simulink model "varParam_laplace"  (R2022b)
settings: Solver=VariableStepAuto  StartTime=0.0  StopTime=10.0  MaxStep=1e-3  MinStep=1e-4  RelTol=1e-3
settings Model: Creator=yeyi5  LastModifiedBy=yeyi5
settings DataIOCC: ReturnWorkspaceOutputs=off

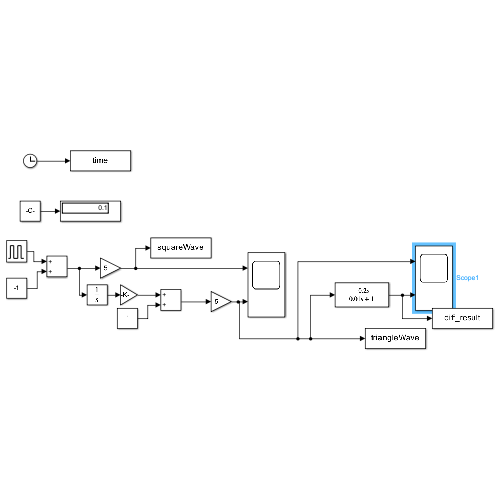
[thumbnail: Simulink's stored preview of the top-level diagram]
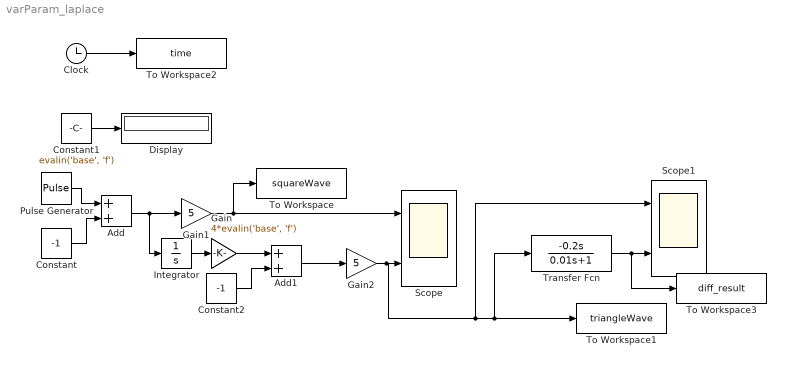
== system varParam_laplace ==
  Add : Sum
  Add1 : Sum
  Clock : Clock
  Constant : Constant  Value=-1
  Constant1 : Constant  Value=evalin('base', 'f')
  Constant2 : Constant  Value=-1
  Display : Display
  Gain : Gain  Gain=4*evalin('base', 'f')
  Gain1 : Gain  Gain=5
  Gain2 : Gain  Gain=5
  Integrator : Integrator
  Pulse Generator : DiscretePulseGenerator  PulseType=Time based  Amplitude=2  Period=evalin('base', '1/f')  PulseWidth=50
  Scope : Scope  NumInputPorts=2
  Scope1 : Scope  NumInputPorts=2
  To Workspace : ToWorkspace  VariableName=squareWave  SampleTime=-1
  To Workspace1 : ToWorkspace  VariableName=triangleWave  SampleTime=-1
  To Workspace2 : ToWorkspace  VariableName=time  SampleTime=-1
  To Workspace3 : ToWorkspace  VariableName=diff_result  SampleTime=-1
  Transfer Fcn : TransferFcn  Numerator=[-0.2, 0]  Denominator=[0.01, 1]
  wires:
  Gain2/1 -> Scope1/1, Transfer Fcn/1, To Workspace1/1, Scope/2
  Constant2/1 -> Add1/2
  Clock/1 -> To Workspace2/1
  Gain1/1 -> To Workspace/1, Scope/1
  Constant1/1 -> Display/1
  Add/1 -> Gain1/1, Integrator/1
  Gain/1 -> Add1/1
  Integrator/1 -> Gain/1
  Pulse Generator/1 -> Add/1
  Constant/1 -> Add/2
  Add1/1 -> Gain2/1
  Transfer Fcn/1 -> To Workspace3/1, Scope1/2
